simulink model "Transitions1_2018a"  (R2018a)
settings: Solver=VariableStepAuto  StartTime=0.0  StopTime=0.1  RelTol=1e-3
settings Model: Creator=BEAR  LastModifiedBy=bzhan

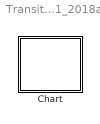
== system Transitions1_2018a ==
  Chart : Stateflow chart  TreatAsAtomicUnit=on

== stateflow chart Transitions1_2018a/Chart ==
  settings: updateMethod=DISCRETE  sampleTime=0.1
  state S
    en: f("enS")
    ex: f("exS")
    state A
      en: f("enA")
      ex: f("exA")
    (default) -> A
  state T
    en: f("enT")
    ex: f("exT")
    state B
      en: f("enB")
      ex: f("exB")
    (default) -> B
  (default) -> S
  A -> B : {f("ca")}/{f("ta")}
  data: s function_input
  function f(s):
    | function f(s)
    |   fprintf(s+"\n");
